simulink model "fuel_v"  (R2019a)
settings: Solver=FixedStepAuto  StartTime=0.0  StopTime=20  FixedStep=1  RelTol=1e-3
model workspace (MAT data in the model file):
  moter_conditionoffvxvvxcvxcvxcvxcvxcvxcvxcvxccvxvxcvxcvxcvx = Simulink.Parameter
  moter_conditionoffvxvvxcvxcvxcvxcvxcvxcvxcvxccvxvxcvxcvxcvx.Value = 0
  moter_conditionoffvxvvxcvxcvxcvxcvxcvxcvxcvxccvxvxcvxcvxcvx.DataType = 'int8'
  moter_conditionoffvxvvxcvxcvxcvxcvxcvxcvxcvxccvxvxcvxcvxcvx.Dimensions = [1 1]
  moter_conditionon = Simulink.Parameter
  moter_conditionon.Value = 1
  moter_conditionon.DataType = 'uint8'
  moter_conditionon.Dimensions = [1 1]
  water_levelhigh = Simulink.Parameter
  water_levelhigh.Value = 9
  water_levelhigh.DataType = 'int8'
  water_levelhigh.Dimensions = [1 1]
  water_levellow = Simulink.Parameter
  water_levellow.Value = 1
  water_levellow.DataType = 'int8'
  water_levellow.Dimensions = [1 1]
settings Model: DataDictionary=DF.sldd  OrderedModelArguments=off  Creator=MY MIND  LastModifiedBy=MY MIND
settings OptimizationCC: DefaultParameterBehavior=Inlined  UseDivisionForNetSlopeComputation=on  EnhancedBackFolding=on  PassReuseOutputArgsAs=Individual arguments  OptimizeBlockOrder=speed  DifferentSizesBufferReuse=on  OptimizationCustomize=off
settings DebuggingCC: SignalInfNanChecking=error  AlgebraicLoopMsg=none  IntegerOverflowMsg=error  ParameterTunabilityLossMsg=error  AssertControl=DisableAll  StrictBusMsg=ErrorOnBusTreatedAsVector  SFUndirectedBroadcastEventsDiag=error
settings SFSimCC: CompileTimeRecursionLimit=0  EnableRuntimeRecursion=off  MATLABDynamicMemAlloc=off
settings RTWCC: SystemTargetFile=ert.tlc  TemplateMakefile=ert_default_tmf  GenerateReport=on  Toolchain=MinGW64 | gmake (64-bit Windows)  IncludeHyperlinkInReport=on  LaunchReport=on  GenerateTraceInfo=on  GenerateTraceReport=on  GenerateTraceReportSl=on  GenerateTraceReportSf=on  GenerateTraceReportEml=on
settings CodeAppCC: ForceParamTrailComments=on  IgnoreCustomStorageClasses=off  OperatorAnnotations=on  SimulinkDataObjDesc=on  SFDataObjDesc=on  MATLABFcnDesc=on  InsertBlockDesc=on
settings ERTTargetCC: TargetLangStandard=C99 (ISO)  UtilityFuncGeneration=Shared location  GenerateSampleERTMain=on  SupportNonFinite=off  ParenthesesLevel=Maximum  CastingMode=Standards  GenerateSharedConstants=off  InlinedParameterPlacement=NonHierarchical  ERTCustomFileTemplate=example_file_process.tlc  EnableSignedLeftShifts=off  EnableSignedRightShifts=off

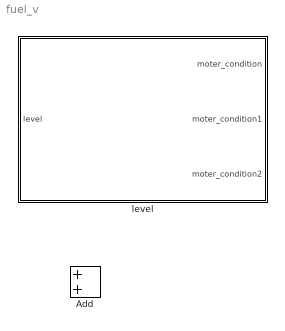
== system fuel_v ==
  Add : Sum
  level : Subsystem  TreatAsAtomicUnit=on

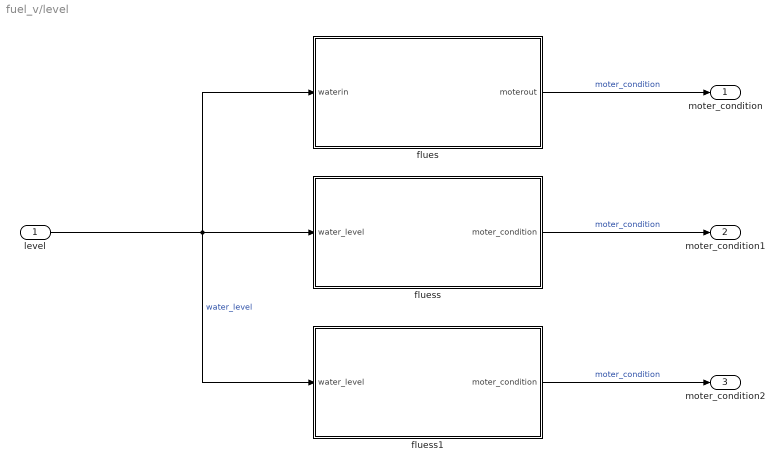
== system fuel_v/level ==
  level : Inport
  flues : Subsystem  TreatAsAtomicUnit=on
  fluess : Stateflow chart  BlockKeywords=__PRM__SERIALIZED__DATA__:Stateflow Chart,Stateflow Diagram  TreatAsAtomicUnit=on
  fluess1 : Stateflow chart  BlockKeywords=__PRM__SERIALIZED__DATA__:Stateflow Chart,Stateflow Diagram  TreatAsAtomicUnit=on
  moter_condition : Outport
  moter_condition1 : Outport  Port=2
  moter_condition2 : Outport  Port=3
  wires:
  level/1 -> flues/1(waterin), fluess/1(water_level), fluess1/1(water_level)  "water_level"
  fluess/1(moter_condition) -> moter_condition1/1  "moter_condition"
  flues/1(moterout) -> moter_condition/1  "moter_condition"
  fluess1/1(moter_condition) -> moter_condition2/1  "moter_condition"

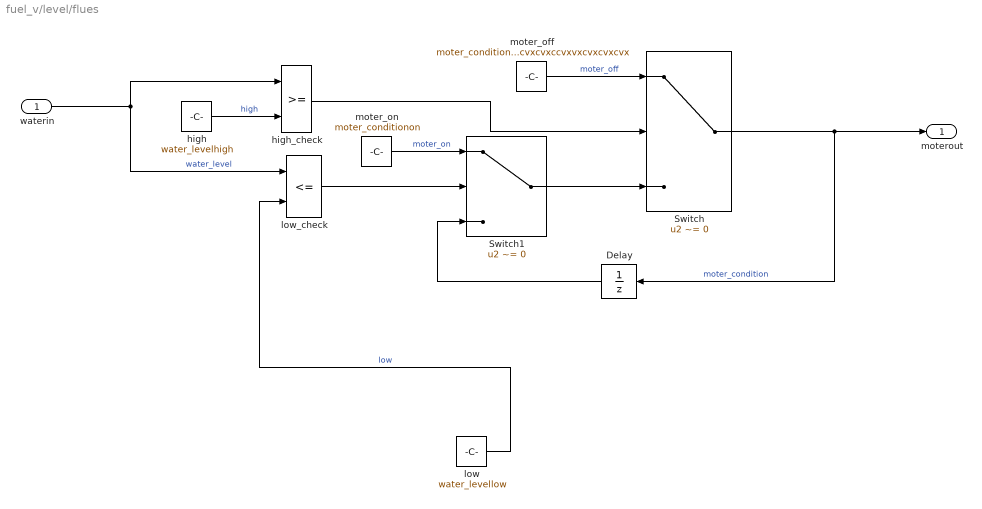
== system fuel_v/level/flues ==
  waterin : Inport
  Delay : UnitDelay  SampleTime=-1  HasFrameUpgradeWarning=on
  Switch : Switch  Criteria=u2 ~= 0
  Switch1 : Switch  Criteria=u2 ~= 0
  high : Constant  Value=water_levelhigh
  high_check : RelationalOperator  OutDataTypeStr=boolean  RndMeth=Simplest
  low : Constant  Value=water_levellow
  low_check : RelationalOperator  Operator=<=  OutDataTypeStr=boolean  RndMeth=Simplest
  moter_off : Constant  Value=moter_conditionoffvxvvxcvxcvxcvxcvxcvxcvxcvxccvxvxcvxcvxcvx
  moter_on : Constant  Value=moter_conditionon
  moterout : Outport
  wires:
  high_check/1 -> Switch/2
  moter_off/1 -> Switch/1  "moter_off"
  Switch1/1 -> Switch/3
  Switch/1 -> Delay/1, moterout/1  "moter_condition"
  low_check/1 -> Switch1/2
  moter_on/1 -> Switch1/1  "moter_on"
  low/1 -> low_check/2  "low"
  high/1 -> high_check/2  "high"
  waterin/1 -> high_check/1, low_check/1  "water_level"
  Delay/1 -> Switch1/3

== stateflow chart fuel_v/level/fluess ==
  state off
    en:
    moter_condition=0;
  state on
    en:
    moter_condition=1;
  (default) -> off
  off -> on : [water_level<=1]
  on -> off : [water_level>=9]
  data: water_level input; moter_condition output

== stateflow chart fuel_v/level/fluess1 ==
  (default) -> (junction 17)
  (junction 17) -> (junction 19) [order 2] : [water_level>=9]
  (junction 17) -> (junction 18) [order 1] : [water_level<=1]
  (junction 19) -> (junction 21) : {moter_condition=0;}
  (junction 18) -> (junction 21) : {moter_condition=1;}
  data: water_level input; moter_condition output
